simulink model "xieboduoji_13fangzhennow"  (R2023a)
settings: Solver=ode4  StartTime=0.0  StopTime=2.2  FixedStep=5e-7  RelTol=1e-3
undefined symbols (not defined in the file or in its folder): magnitude
libraries: simulink x417, spsRMSLib x70, spsCurrentMeasurementLib x32, spsVoltageMeasurementLib x31, powerlib_meascontrol x24, spsFourierLib x21, spsGroundLib x19, spsThreePhasePISectionLineLib x17, spsThreePhaseSeriesRLCBranchLib x14, spsdq0toAlphaBetaZeroLib x13, spsSeriesRLCBranchLib x11, spsUniversalBridgeLib x11
(part 5 of 12)

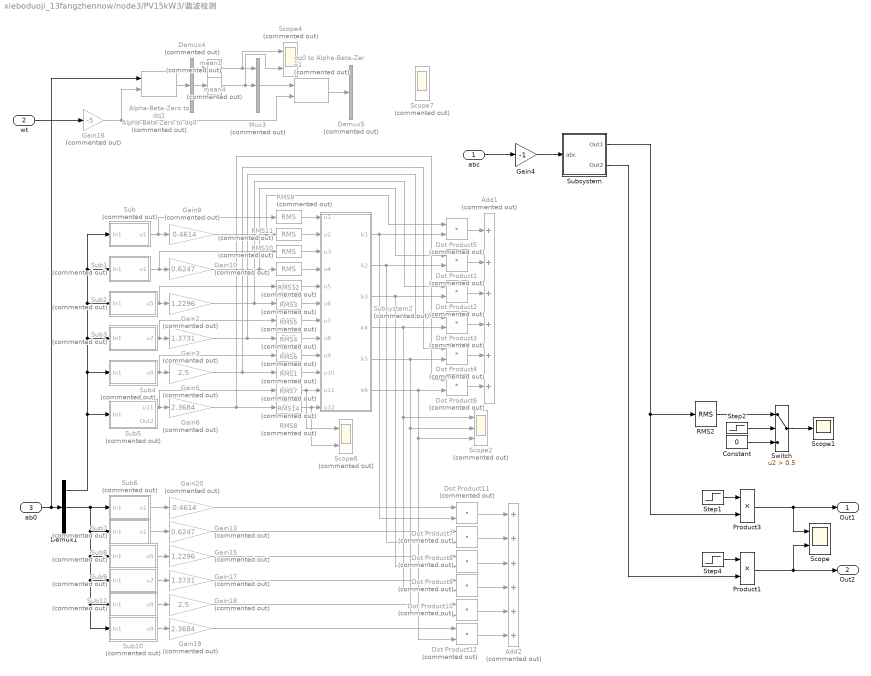
== system xieboduoji_13fangzhennow/node3/PV15kW3/谐波检测 ==
  abc : Inport
  wt : Inport  Port=2
  ab0 : Inport  Port=3
  Add1 : Sum  Commented=on  Inputs=++++++
  Add2 : Sum  Commented=on  Inputs=++++++
  Alpha-Beta-Zero to dq1 : spsAlphaBetaZerotodq0Lib/Alpha-Beta-Zero to dq0  Commented=on  Alignment=Aligned with phase A axis
  Constant : Constant  Value=0
  Demux1 : Demux  Outputs=3
  Demux4 : Demux  Commented=on  Outputs=3
  Demux5 : Demux  Commented=on  Outputs=3
  Dot Product{1..12} (12 alike) : DotProduct  Commented=on  OutDataTypeStr=Inherit: Inherit via internal rule
  Gain10 : Gain  Commented=on  Gain=0.6247
  Gain13 : Gain  Commented=on  Gain=0.6247
  Gain15 : Gain  Commented=on  Gain=1.2296
  Gain16 : Gain  Commented=on  Gain=-5
  Gain17 : Gain  Commented=on  Gain=1.3731
  Gain18 : Gain  Commented=on  Gain=2.5
  Gain19 : Gain  Commented=on  Gain=2.3684
  Gain2 : Gain  Commented=on  Gain=1.2296
  Gain20 : Gain  Commented=on  Gain=0.4614
  Gain3 : Gain  Commented=on  Gain=1.3731
  Gain4 : Gain  Gain=-1
  Gain5 : Gain  Commented=on  Gain=2.5
  Gain6 : Gain  Commented=on  Gain=2.3684
  Gain9 : Gain  Commented=on  Gain=0.4614
  Mux3 : Mux  Commented=on  Inputs=3
  Product1 : Product
  Product3 : Product
  RMS{1,3..12,14} (12 alike) : spsRMSLib/RMS  Commented=on  TrueRMS=on  Freq=100  RMSInit=0  Ts=5e-5
  RMS2 : spsRMSLib/RMS  TrueRMS=on  Freq=50  RMSInit=0  Ts=5e-5
  Scope : Scope  NumInputPorts=2
  Scope1 : Scope
  Scope2 : Scope  Commented=on  NumInputPorts=3
  Scope4 : Scope  Commented=on  NumInputPorts=2
  Scope6 : Scope  Commented=on  NumInputPorts=2
  Scope7 : Scope  Commented=on  NumInputPorts=2
  Step1 : Step  After=-1  SampleTime=0
  Step2 : Step  SampleTime=0
  Step4 : Step  After=-1  SampleTime=0
  Sub : Subsystem  Commented=on
  Sub1 : Subsystem  Commented=on
  Sub10 : Subsystem  Commented=on
  Sub12 : Subsystem  Commented=on
  Sub2 : Subsystem  Commented=on
  Sub3 : Subsystem  Commented=on
  Sub4 : Subsystem  Commented=on
  Sub5 : Subsystem  Commented=on
  Sub6 : Subsystem  Commented=on
  Sub7 : Subsystem  Commented=on
  Sub8 : Subsystem  Commented=on
  Sub9 : Subsystem  Commented=on
  Subsystem : Subsystem
  Subsystem2 : Subsystem  Commented=on
  Switch : Switch  Criteria=u2 > Threshold  Threshold=0.5  SaturateOnIntegerOverflow=off  InputSameDT=off
  dq0 to Alpha-Beta-Zero1 : spsdq0toAlphaBetaZeroLib/dq0 to Alpha-Beta-Zero  Commented=on  Alignment=Aligned with phase A axis
  mean1 : spsMeanLib/Mean  Commented=on  Freq=50  Vinit=0  Ts=5e-5
  mean4 : spsMeanLib/Mean  Commented=on  Freq=50  Vinit=0  Ts=5e-5
  Out1 : Outport
  Out2 : Outport  Port=2
  wires:
  abc/1 -> Gain4/1
  Step1/1 -> Product3/1
  Step2/1 -> Switch/2
  Constant/1 -> Switch/3
  Switch/1 -> Scope1/1
  Sub5/1(u11) -> RMS14/1, Gain6/1
  Sub4/1(u9) -> Gain5/1, RMS1/1
  Sub3/1(u7) -> RMS4/1, Gain3/1
  Sub2/1(u5) -> RMS3/1, Gain2/1
  Demux1/1 -> Sub/1(In1), Sub1/1(In1), Sub2/1(In1), Sub3/1(In1), Sub4/1(In1), Sub5/1(In1)
  Sub1/1(u1) -> RMS10/1, Gain10/1
  Subsystem2/1(k1) -> Dot Product5/2, Dot Product11/2
  Subsystem2/2(k2) -> Dot Product7/2, Dot Product1/2
  Subsystem2/3(k3) -> Dot Product8/2, Dot Product2/2
  Subsystem2/4(k4) -> Scope2/1, Dot Product9/2, Dot Product3/2
  Subsystem2/5(k5) -> Dot Product10/2, Scope2/2, Dot Product4/2
  Sub8/1(u5) -> Gain15/1
  Sub9/1(u7) -> Gain17/1
  Sub12/1(u9) -> Gain18/1
  Demux1/2 -> Sub6/1(In1), Sub7/1(In1), Sub8/1(In1), Sub9/1(In1), Sub10/1(In1), Sub12/1(In1)
  Dot Product12/1 -> Add2/6
  Dot Product10/1 -> Add2/5
  Gain9/1 -> RMS11/1, Dot Product5/1
  Gain2/1 -> RMS5/1, Dot Product2/1
  Gain3/1 -> Dot Product3/1, RMS6/1
  Gain5/1 -> RMS7/1, Dot Product4/1
  Gain6/1 -> Dot Product6/1, RMS8/1
  Gain20/1 -> Dot Product11/1
  Gain13/1 -> Dot Product7/1
  Gain15/1 -> Dot Product8/1
  Gain17/1 -> Dot Product9/1
  Gain18/1 -> Dot Product10/1
  Gain19/1 -> Dot Product12/1
  RMS2/1 -> Switch/1
  RMS7/1 -> Subsystem2/10(u10)
  RMS8/1 -> Scope6/2, Subsystem2/12(u12)
  Gain10/1 -> RMS12/1, Dot Product1/1
  RMS1/1 -> Subsystem2/9(u9)
  RMS14/1 -> Subsystem2/11(u11), Scope6/1
  Dot Product6/1 -> Add1/6
  Dot Product4/1 -> Add1/5
  RMS10/1 -> Subsystem2/3(u3)
  RMS3/1 -> Subsystem2/5(u5)
  RMS5/1 -> Subsystem2/6(u6)
  RMS4/1 -> Subsystem2/7(u7)
  RMS6/1 -> Subsystem2/8(u8)
  Step4/1 -> Product1/1
  Product1/1 -> Scope/2, Out2/1
  Product3/1 -> Scope/1, Out1/1
  Dot Product2/1 -> Add1/3
  Dot Product3/1 -> Add1/4
  Subsystem2/6(k6) -> Scope2/3, Dot Product12/2, Dot Product6/2
  Dot Product8/1 -> Add2/3
  Dot Product9/1 -> Add2/4
  RMS9/1 -> Subsystem2/1(u1)
  Dot Product5/1 -> Add1/1
  Dot Product1/1 -> Add1/2
  Dot Product11/1 -> Add2/1
  Dot Product7/1 -> Add2/2
  RMS11/1 -> Subsystem2/2(u2)
  RMS12/1 -> Subsystem2/4(u4)
  mean1/1 -> Mux3/2, Scope4/2
  mean4/1 -> Mux3/1, Scope4/1
  dq0 to Alpha-Beta-Zero1/1 -> Demux5/1
  Mux3/1 -> dq0 to Alpha-Beta-Zero1/1
  Demux4/2 -> mean1/1
  Demux4/1 -> mean4/1
  Alpha-Beta-Zero to dq1/1 -> Demux4/1
  wt/1 -> Gain16/1
  Gain16/1 -> Alpha-Beta-Zero to dq1/2, dq0 to Alpha-Beta-Zero1/2
  ab0/1 -> Alpha-Beta-Zero to dq1/1, Demux1/1
  Sub/1(u1) -> RMS9/1, Gain9/1
  Sub6/1(u1) -> Gain20/1
  Sub7/1(u1) -> Gain13/1
  Sub10/1(u9) -> Gain19/1
  Gain4/1 -> Subsystem/1(abc)
  Subsystem/1(Out1) -> RMS2/1, Product3/2
  Subsystem/2(Out2) -> Product1/2

== system xieboduoji_13fangzhennow/node3/Subsystem1/RMS1 ==
  u1 : Inport
  u3 : Inport  Port=2
  u4 : Inport  Port=3
  u5 : Inport  Port=4
  u6 : Inport  Port=5
  u2 : Inport  Port=6
  Trigger : TriggerPort  VariantControl=(inherit)
  Scope : Scope  Commented=on
  Scope1 : Scope  Commented=on
  xunidiandao : MATLAB Function  TreatAsAtomicUnit=on
  k1 : Outport  VectorParamsAs1DForOutWhenUnconnected=off
  k2 : Outport  Port=2  VectorParamsAs1DForOutWhenUnconnected=off
  k3 : Outport  Port=3  VectorParamsAs1DForOutWhenUnconnected=off
  k4 : Outport  Port=4  VectorParamsAs1DForOutWhenUnconnected=off
  k5 : Outport  Port=5  VectorParamsAs1DForOutWhenUnconnected=off
  k6 : Outport  Port=6  VectorParamsAs1DForOutWhenUnconnected=off
  k7 : Outport  Port=7  VectorParamsAs1DForOutWhenUnconnected=off
  k8 : Outport  Port=8  VectorParamsAs1DForOutWhenUnconnected=off
  k9 : Outport  Port=9  VectorParamsAs1DForOutWhenUnconnected=off
  k10 : Outport  Port=10  VectorParamsAs1DForOutWhenUnconnected=off
  k11 : Outport  Port=11  VectorParamsAs1DForOutWhenUnconnected=off
  k12 : Outport  Port=12  VectorParamsAs1DForOutWhenUnconnected=off
  wires:
  xunidiandao/13(x) -> Scope/1
  u3/1 -> xunidiandao/2(u2)
  u4/1 -> xunidiandao/3(u3)
  u5/1 -> xunidiandao/4(u4)
  u6/1 -> xunidiandao/5(u5)
  u2/1 -> xunidiandao/6(u6)
  u1/1 -> xunidiandao/1(u1)
  xunidiandao/12(y66) -> k12/1
  xunidiandao/11(y6) -> k11/1
  xunidiandao/10(y55) -> k10/1
  xunidiandao/9(y5) -> k9/1
  xunidiandao/8(y44) -> k8/1
  xunidiandao/7(y4) -> k7/1
  xunidiandao/6(y33) -> k6/1
  xunidiandao/5(y3) -> k5/1
  xunidiandao/4(y22) -> k4/1
  xunidiandao/3(y2) -> k3/1
  xunidiandao/2(y11) -> k2/1
  xunidiandao/1(y1) -> k1/1, Scope1/1

== system xieboduoji_13fangzhennow/node3/Subsystem2/RMS1 ==
  u1 : Inport
  u3 : Inport  Port=2
  u4 : Inport  Port=3
  u5 : Inport  Port=4
  u6 : Inport  Port=5
  u2 : Inport  Port=6
  Trigger : TriggerPort  VariantControl=(inherit)
  Scope : Scope  Commented=on
  Scope1 : Scope  Commented=on
  xunidiandao : MATLAB Function  TreatAsAtomicUnit=on
  k1 : Outport  VectorParamsAs1DForOutWhenUnconnected=off
  k2 : Outport  Port=2  VectorParamsAs1DForOutWhenUnconnected=off
  k3 : Outport  Port=3  VectorParamsAs1DForOutWhenUnconnected=off
  k4 : Outport  Port=4  VectorParamsAs1DForOutWhenUnconnected=off
  k5 : Outport  Port=5  VectorParamsAs1DForOutWhenUnconnected=off
  k6 : Outport  Port=6  VectorParamsAs1DForOutWhenUnconnected=off
  k7 : Outport  Port=7  VectorParamsAs1DForOutWhenUnconnected=off
  k8 : Outport  Port=8  VectorParamsAs1DForOutWhenUnconnected=off
  k9 : Outport  Port=9  VectorParamsAs1DForOutWhenUnconnected=off
  k10 : Outport  Port=10  VectorParamsAs1DForOutWhenUnconnected=off
  k11 : Outport  Port=11  VectorParamsAs1DForOutWhenUnconnected=off
  k12 : Outport  Port=12  VectorParamsAs1DForOutWhenUnconnected=off
  wires:
  xunidiandao/1(y1) -> Scope1/1, k1/1
  xunidiandao/2(y11) -> k2/1
  xunidiandao/3(y2) -> k3/1
  xunidiandao/4(y22) -> k4/1
  xunidiandao/5(y3) -> k5/1
  xunidiandao/6(y33) -> k6/1
  xunidiandao/7(y4) -> k7/1
  xunidiandao/8(y44) -> k8/1
  xunidiandao/9(y5) -> k9/1
  xunidiandao/10(y55) -> k10/1
  xunidiandao/11(y6) -> k11/1
  xunidiandao/12(y66) -> k12/1
  u1/1 -> xunidiandao/1(u1)
  u2/1 -> xunidiandao/6(u6)
  u6/1 -> xunidiandao/5(u5)
  u5/1 -> xunidiandao/4(u4)
  u4/1 -> xunidiandao/3(u3)
  u3/1 -> xunidiandao/2(u2)
  xunidiandao/13(x) -> Scope/1

== system xieboduoji_13fangzhennow/node3/谐波源/Subsystem1 ==
  u1 : Inport
  u3 : Inport  Port=2
  u4 : Inport  Port=3
  u5 : Inport  Port=4
  u6 : Inport  Port=5
  u2 : Inport  Port=6
  Pul : DiscretePulseGenerator  PulseType=Time based  Period=5e-5  PulseWidth=40
  RMS1 : Subsystem  TreatAsAtomicUnit=on
  k1 : Outport  VectorParamsAs1DForOutWhenUnconnected=off
  k2 : Outport  Port=2  VectorParamsAs1DForOutWhenUnconnected=off
  k3 : Outport  Port=3  VectorParamsAs1DForOutWhenUnconnected=off
  k4 : Outport  Port=4  VectorParamsAs1DForOutWhenUnconnected=off
  k5 : Outport  Port=5  VectorParamsAs1DForOutWhenUnconnected=off
  k6 : Outport  Port=6  VectorParamsAs1DForOutWhenUnconnected=off
  k7 : Outport  Port=7  VectorParamsAs1DForOutWhenUnconnected=off
  k8 : Outport  Port=8  VectorParamsAs1DForOutWhenUnconnected=off
  k9 : Outport  Port=9  VectorParamsAs1DForOutWhenUnconnected=off
  k10 : Outport  Port=10  VectorParamsAs1DForOutWhenUnconnected=off
  k11 : Outport  Port=11  VectorParamsAs1DForOutWhenUnconnected=off
  k12 : Outport  Port=12  VectorParamsAs1DForOutWhenUnconnected=off
  wires:
  u2/1 -> RMS1/6(u2)
  u6/1 -> RMS1/5(u6)
  u5/1 -> RMS1/4(u5)
  u4/1 -> RMS1/3(u4)
  u3/1 -> RMS1/2(u3)
  u1/1 -> RMS1/1(u1)
  RMS1/12(k12) -> k12/1
  RMS1/11(k11) -> k11/1
  RMS1/10(k10) -> k10/1
  RMS1/9(k9) -> k9/1
  RMS1/8(k8) -> k8/1
  RMS1/7(k7) -> k7/1
  RMS1/6(k6) -> k6/1
  RMS1/5(k5) -> k5/1
  RMS1/4(k4) -> k4/1
  RMS1/3(k3) -> k3/1
  RMS1/2(k2) -> k2/1
  RMS1/1(k1) -> k1/1
  Pul/1 -> RMS1/Trigger

== system xieboduoji_13fangzhennow/node3/谐波源/Subsystem2 ==
  u1 : Inport
  u3 : Inport  Port=2
  u4 : Inport  Port=3
  u5 : Inport  Port=4
  u6 : Inport  Port=5
  u2 : Inport  Port=6
  Pul : DiscretePulseGenerator  PulseType=Time based  Period=5e-5  PulseWidth=40
  RMS1 : Subsystem  TreatAsAtomicUnit=on
  k1 : Outport  VectorParamsAs1DForOutWhenUnconnected=off
  k2 : Outport  Port=2  VectorParamsAs1DForOutWhenUnconnected=off
  k3 : Outport  Port=3  VectorParamsAs1DForOutWhenUnconnected=off
  k4 : Outport  Port=4  VectorParamsAs1DForOutWhenUnconnected=off
  k5 : Outport  Port=5  VectorParamsAs1DForOutWhenUnconnected=off
  k6 : Outport  Port=6  VectorParamsAs1DForOutWhenUnconnected=off
  k7 : Outport  Port=7  VectorParamsAs1DForOutWhenUnconnected=off
  k8 : Outport  Port=8  VectorParamsAs1DForOutWhenUnconnected=off
  k9 : Outport  Port=9  VectorParamsAs1DForOutWhenUnconnected=off
  k10 : Outport  Port=10  VectorParamsAs1DForOutWhenUnconnected=off
  k11 : Outport  Port=11  VectorParamsAs1DForOutWhenUnconnected=off
  k12 : Outport  Port=12  VectorParamsAs1DForOutWhenUnconnected=off
  wires:
  Pul/1 -> RMS1/Trigger
  RMS1/1(k1) -> k1/1
  RMS1/2(k2) -> k2/1
  RMS1/3(k3) -> k3/1
  RMS1/4(k4) -> k4/1
  RMS1/5(k5) -> k5/1
  RMS1/6(k6) -> k6/1
  RMS1/7(k7) -> k7/1
  RMS1/8(k8) -> k8/1
  RMS1/9(k9) -> k9/1
  RMS1/10(k10) -> k10/1
  RMS1/11(k11) -> k11/1
  RMS1/12(k12) -> k12/1
  u1/1 -> RMS1/1(u1)
  u3/1 -> RMS1/2(u3)
  u4/1 -> RMS1/3(u4)
  u5/1 -> RMS1/4(u5)
  u6/1 -> RMS1/5(u6)
  u2/1 -> RMS1/6(u2)

== system xieboduoji_13fangzhennow/node4/Subsystem1/RMS1 ==
  u1 : Inport
  u3 : Inport  Port=2
  u4 : Inport  Port=3
  u5 : Inport  Port=4
  u6 : Inport  Port=5
  u2 : Inport  Port=6
  Trigger : TriggerPort  VariantControl=(inherit)
  Scope : Scope  Commented=on
  Scope1 : Scope  Commented=on
  xunidiandao : MATLAB Function  TreatAsAtomicUnit=on
  k1 : Outport  VectorParamsAs1DForOutWhenUnconnected=off
  k2 : Outport  Port=2  VectorParamsAs1DForOutWhenUnconnected=off
  k3 : Outport  Port=3  VectorParamsAs1DForOutWhenUnconnected=off
  k4 : Outport  Port=4  VectorParamsAs1DForOutWhenUnconnected=off
  k5 : Outport  Port=5  VectorParamsAs1DForOutWhenUnconnected=off
  k6 : Outport  Port=6  VectorParamsAs1DForOutWhenUnconnected=off
  k7 : Outport  Port=7  VectorParamsAs1DForOutWhenUnconnected=off
  k8 : Outport  Port=8  VectorParamsAs1DForOutWhenUnconnected=off
  k9 : Outport  Port=9  VectorParamsAs1DForOutWhenUnconnected=off
  k10 : Outport  Port=10  VectorParamsAs1DForOutWhenUnconnected=off
  k11 : Outport  Port=11  VectorParamsAs1DForOutWhenUnconnected=off
  k12 : Outport  Port=12  VectorParamsAs1DForOutWhenUnconnected=off
  wires:
  xunidiandao/13(x) -> Scope/1
  u3/1 -> xunidiandao/2(u2)
  u4/1 -> xunidiandao/3(u3)
  u5/1 -> xunidiandao/4(u4)
  u6/1 -> xunidiandao/5(u5)
  u2/1 -> xunidiandao/6(u6)
  u1/1 -> xunidiandao/1(u1)
  xunidiandao/12(y66) -> k12/1
  xunidiandao/11(y6) -> k11/1
  xunidiandao/10(y55) -> k10/1
  xunidiandao/9(y5) -> k9/1
  xunidiandao/8(y44) -> k8/1
  xunidiandao/7(y4) -> k7/1
  xunidiandao/6(y33) -> k6/1
  xunidiandao/5(y3) -> k5/1
  xunidiandao/4(y22) -> k4/1
  xunidiandao/3(y2) -> k3/1
  xunidiandao/2(y11) -> k2/1
  xunidiandao/1(y1) -> k1/1, Scope1/1

== system xieboduoji_13fangzhennow/node4/Subsystem2/RMS1 ==
  u1 : Inport
  u3 : Inport  Port=2
  u4 : Inport  Port=3
  u5 : Inport  Port=4
  u6 : Inport  Port=5
  u2 : Inport  Port=6
  Trigger : TriggerPort  VariantControl=(inherit)
  Scope : Scope  Commented=on
  Scope1 : Scope  Commented=on
  xunidiandao : MATLAB Function  TreatAsAtomicUnit=on
  k1 : Outport  VectorParamsAs1DForOutWhenUnconnected=off
  k2 : Outport  Port=2  VectorParamsAs1DForOutWhenUnconnected=off
  k3 : Outport  Port=3  VectorParamsAs1DForOutWhenUnconnected=off
  k4 : Outport  Port=4  VectorParamsAs1DForOutWhenUnconnected=off
  k5 : Outport  Port=5  VectorParamsAs1DForOutWhenUnconnected=off
  k6 : Outport  Port=6  VectorParamsAs1DForOutWhenUnconnected=off
  k7 : Outport  Port=7  VectorParamsAs1DForOutWhenUnconnected=off
  k8 : Outport  Port=8  VectorParamsAs1DForOutWhenUnconnected=off
  k9 : Outport  Port=9  VectorParamsAs1DForOutWhenUnconnected=off
  k10 : Outport  Port=10  VectorParamsAs1DForOutWhenUnconnected=off
  k11 : Outport  Port=11  VectorParamsAs1DForOutWhenUnconnected=off
  k12 : Outport  Port=12  VectorParamsAs1DForOutWhenUnconnected=off
  wires:
  xunidiandao/1(y1) -> Scope1/1, k1/1
  xunidiandao/2(y11) -> k2/1
  xunidiandao/3(y2) -> k3/1
  xunidiandao/4(y22) -> k4/1
  xunidiandao/5(y3) -> k5/1
  xunidiandao/6(y33) -> k6/1
  xunidiandao/7(y4) -> k7/1
  xunidiandao/8(y44) -> k8/1
  xunidiandao/9(y5) -> k9/1
  xunidiandao/10(y55) -> k10/1
  xunidiandao/11(y6) -> k11/1
  xunidiandao/12(y66) -> k12/1
  u1/1 -> xunidiandao/1(u1)
  u2/1 -> xunidiandao/6(u6)
  u6/1 -> xunidiandao/5(u5)
  u5/1 -> xunidiandao/4(u4)
  u4/1 -> xunidiandao/3(u3)
  u3/1 -> xunidiandao/2(u2)
  xunidiandao/13(x) -> Scope/1

== system xieboduoji_13fangzhennow/node4/谐波源/Subsystem1 ==
  u1 : Inport
  u3 : Inport  Port=2
  u4 : Inport  Port=3
  u5 : Inport  Port=4
  u6 : Inport  Port=5
  u2 : Inport  Port=6
  Pul : DiscretePulseGenerator  PulseType=Time based  Period=5e-5  PulseWidth=40
  RMS1 : Subsystem  TreatAsAtomicUnit=on
  k1 : Outport  VectorParamsAs1DForOutWhenUnconnected=off
  k2 : Outport  Port=2  VectorParamsAs1DForOutWhenUnconnected=off
  k3 : Outport  Port=3  VectorParamsAs1DForOutWhenUnconnected=off
  k4 : Outport  Port=4  VectorParamsAs1DForOutWhenUnconnected=off
  k5 : Outport  Port=5  VectorParamsAs1DForOutWhenUnconnected=off
  k6 : Outport  Port=6  VectorParamsAs1DForOutWhenUnconnected=off
  k7 : Outport  Port=7  VectorParamsAs1DForOutWhenUnconnected=off
  k8 : Outport  Port=8  VectorParamsAs1DForOutWhenUnconnected=off
  k9 : Outport  Port=9  VectorParamsAs1DForOutWhenUnconnected=off
  k10 : Outport  Port=10  VectorParamsAs1DForOutWhenUnconnected=off
  k11 : Outport  Port=11  VectorParamsAs1DForOutWhenUnconnected=off
  k12 : Outport  Port=12  VectorParamsAs1DForOutWhenUnconnected=off
  wires:
  u2/1 -> RMS1/6(u2)
  u6/1 -> RMS1/5(u6)
  u5/1 -> RMS1/4(u5)
  u4/1 -> RMS1/3(u4)
  u3/1 -> RMS1/2(u3)
  u1/1 -> RMS1/1(u1)
  RMS1/12(k12) -> k12/1
  RMS1/11(k11) -> k11/1
  RMS1/10(k10) -> k10/1
  RMS1/9(k9) -> k9/1
  RMS1/8(k8) -> k8/1
  RMS1/7(k7) -> k7/1
  RMS1/6(k6) -> k6/1
  RMS1/5(k5) -> k5/1
  RMS1/4(k4) -> k4/1
  RMS1/3(k3) -> k3/1
  RMS1/2(k2) -> k2/1
  RMS1/1(k1) -> k1/1
  Pul/1 -> RMS1/Trigger

== system xieboduoji_13fangzhennow/node4/谐波源/Subsystem2 ==
  u1 : Inport
  u3 : Inport  Port=2
  u4 : Inport  Port=3
  u5 : Inport  Port=4
  u6 : Inport  Port=5
  u2 : Inport  Port=6
  Pul : DiscretePulseGenerator  PulseType=Time based  Period=5e-5  PulseWidth=40
  RMS1 : Subsystem  TreatAsAtomicUnit=on
  k1 : Outport  VectorParamsAs1DForOutWhenUnconnected=off
  k2 : Outport  Port=2  VectorParamsAs1DForOutWhenUnconnected=off
  k3 : Outport  Port=3  VectorParamsAs1DForOutWhenUnconnected=off
  k4 : Outport  Port=4  VectorParamsAs1DForOutWhenUnconnected=off
  k5 : Outport  Port=5  VectorParamsAs1DForOutWhenUnconnected=off
  k6 : Outport  Port=6  VectorParamsAs1DForOutWhenUnconnected=off
  k7 : Outport  Port=7  VectorParamsAs1DForOutWhenUnconnected=off
  k8 : Outport  Port=8  VectorParamsAs1DForOutWhenUnconnected=off
  k9 : Outport  Port=9  VectorParamsAs1DForOutWhenUnconnected=off
  k10 : Outport  Port=10  VectorParamsAs1DForOutWhenUnconnected=off
  k11 : Outport  Port=11  VectorParamsAs1DForOutWhenUnconnected=off
  k12 : Outport  Port=12  VectorParamsAs1DForOutWhenUnconnected=off
  wires:
  Pul/1 -> RMS1/Trigger
  RMS1/1(k1) -> k1/1
  RMS1/2(k2) -> k2/1
  RMS1/3(k3) -> k3/1
  RMS1/4(k4) -> k4/1
  RMS1/5(k5) -> k5/1
  RMS1/6(k6) -> k6/1
  RMS1/7(k7) -> k7/1
  RMS1/8(k8) -> k8/1
  RMS1/9(k9) -> k9/1
  RMS1/10(k10) -> k10/1
  RMS1/11(k11) -> k11/1
  RMS1/12(k12) -> k12/1
  u1/1 -> RMS1/1(u1)
  u3/1 -> RMS1/2(u3)
  u4/1 -> RMS1/3(u4)
  u5/1 -> RMS1/4(u5)
  u6/1 -> RMS1/5(u6)
  u2/1 -> RMS1/6(u2)

== system xieboduoji_13fangzhennow/node5/Subsystem1/RMS1 ==
  u1 : Inport
  u3 : Inport  Port=2
  u4 : Inport  Port=3
  u5 : Inport  Port=4
  u6 : Inport  Port=5
  u2 : Inport  Port=6
  Trigger : TriggerPort  VariantControl=(inherit)
  Scope : Scope  Commented=on
  Scope1 : Scope  Commented=on
  xunidiandao : MATLAB Function  TreatAsAtomicUnit=on
  k1 : Outport  VectorParamsAs1DForOutWhenUnconnected=off
  k2 : Outport  Port=2  VectorParamsAs1DForOutWhenUnconnected=off
  k3 : Outport  Port=3  VectorParamsAs1DForOutWhenUnconnected=off
  k4 : Outport  Port=4  VectorParamsAs1DForOutWhenUnconnected=off
  k5 : Outport  Port=5  VectorParamsAs1DForOutWhenUnconnected=off
  k6 : Outport  Port=6  VectorParamsAs1DForOutWhenUnconnected=off
  k7 : Outport  Port=7  VectorParamsAs1DForOutWhenUnconnected=off
  k8 : Outport  Port=8  VectorParamsAs1DForOutWhenUnconnected=off
  k9 : Outport  Port=9  VectorParamsAs1DForOutWhenUnconnected=off
  k10 : Outport  Port=10  VectorParamsAs1DForOutWhenUnconnected=off
  k11 : Outport  Port=11  VectorParamsAs1DForOutWhenUnconnected=off
  k12 : Outport  Port=12  VectorParamsAs1DForOutWhenUnconnected=off
  wires:
  xunidiandao/13(x) -> Scope/1
  u3/1 -> xunidiandao/2(u2)
  u4/1 -> xunidiandao/3(u3)
  u5/1 -> xunidiandao/4(u4)
  u6/1 -> xunidiandao/5(u5)
  u2/1 -> xunidiandao/6(u6)
  u1/1 -> xunidiandao/1(u1)
  xunidiandao/12(y66) -> k12/1
  xunidiandao/11(y6) -> k11/1
  xunidiandao/10(y55) -> k10/1
  xunidiandao/9(y5) -> k9/1
  xunidiandao/8(y44) -> k8/1
  xunidiandao/7(y4) -> k7/1
  xunidiandao/6(y33) -> k6/1
  xunidiandao/5(y3) -> k5/1
  xunidiandao/4(y22) -> k4/1
  xunidiandao/3(y2) -> k3/1
  xunidiandao/2(y11) -> k2/1
  xunidiandao/1(y1) -> k1/1, Scope1/1

== system xieboduoji_13fangzhennow/node5/Subsystem2/RMS1 ==
  u1 : Inport
  u3 : Inport  Port=2
  u4 : Inport  Port=3
  u5 : Inport  Port=4
  u6 : Inport  Port=5
  u2 : Inport  Port=6
  Trigger : TriggerPort  VariantControl=(inherit)
  Scope : Scope  Commented=on
  Scope1 : Scope  Commented=on
  xunidiandao : MATLAB Function  TreatAsAtomicUnit=on
  k1 : Outport  VectorParamsAs1DForOutWhenUnconnected=off
  k2 : Outport  Port=2  VectorParamsAs1DForOutWhenUnconnected=off
  k3 : Outport  Port=3  VectorParamsAs1DForOutWhenUnconnected=off
  k4 : Outport  Port=4  VectorParamsAs1DForOutWhenUnconnected=off
  k5 : Outport  Port=5  VectorParamsAs1DForOutWhenUnconnected=off
  k6 : Outport  Port=6  VectorParamsAs1DForOutWhenUnconnected=off
  k7 : Outport  Port=7  VectorParamsAs1DForOutWhenUnconnected=off
  k8 : Outport  Port=8  VectorParamsAs1DForOutWhenUnconnected=off
  k9 : Outport  Port=9  VectorParamsAs1DForOutWhenUnconnected=off
  k10 : Outport  Port=10  VectorParamsAs1DForOutWhenUnconnected=off
  k11 : Outport  Port=11  VectorParamsAs1DForOutWhenUnconnected=off
  k12 : Outport  Port=12  VectorParamsAs1DForOutWhenUnconnected=off
  wires:
  xunidiandao/1(y1) -> Scope1/1, k1/1
  xunidiandao/2(y11) -> k2/1
  xunidiandao/3(y2) -> k3/1
  xunidiandao/4(y22) -> k4/1
  xunidiandao/5(y3) -> k5/1
  xunidiandao/6(y33) -> k6/1
  xunidiandao/7(y4) -> k7/1
  xunidiandao/8(y44) -> k8/1
  xunidiandao/9(y5) -> k9/1
  xunidiandao/10(y55) -> k10/1
  xunidiandao/11(y6) -> k11/1
  xunidiandao/12(y66) -> k12/1
  u1/1 -> xunidiandao/1(u1)
  u2/1 -> xunidiandao/6(u6)
  u6/1 -> xunidiandao/5(u5)
  u5/1 -> xunidiandao/4(u4)
  u4/1 -> xunidiandao/3(u3)
  u3/1 -> xunidiandao/2(u2)
  xunidiandao/13(x) -> Scope/1

== system xieboduoji_13fangzhennow/node5/谐波源/Subsystem1 ==
  u1 : Inport
  u3 : Inport  Port=2
  u4 : Inport  Port=3
  u5 : Inport  Port=4
  u6 : Inport  Port=5
  u2 : Inport  Port=6
  Pul : DiscretePulseGenerator  PulseType=Time based  Period=5e-5  PulseWidth=40
  RMS1 : Subsystem  TreatAsAtomicUnit=on
  k1 : Outport  VectorParamsAs1DForOutWhenUnconnected=off
  k2 : Outport  Port=2  VectorParamsAs1DForOutWhenUnconnected=off
  k3 : Outport  Port=3  VectorParamsAs1DForOutWhenUnconnected=off
  k4 : Outport  Port=4  VectorParamsAs1DForOutWhenUnconnected=off
  k5 : Outport  Port=5  VectorParamsAs1DForOutWhenUnconnected=off
  k6 : Outport  Port=6  VectorParamsAs1DForOutWhenUnconnected=off
  k7 : Outport  Port=7  VectorParamsAs1DForOutWhenUnconnected=off
  k8 : Outport  Port=8  VectorParamsAs1DForOutWhenUnconnected=off
  k9 : Outport  Port=9  VectorParamsAs1DForOutWhenUnconnected=off
  k10 : Outport  Port=10  VectorParamsAs1DForOutWhenUnconnected=off
  k11 : Outport  Port=11  VectorParamsAs1DForOutWhenUnconnected=off
  k12 : Outport  Port=12  VectorParamsAs1DForOutWhenUnconnected=off
  wires:
  u2/1 -> RMS1/6(u2)
  u6/1 -> RMS1/5(u6)
  u5/1 -> RMS1/4(u5)
  u4/1 -> RMS1/3(u4)
  u3/1 -> RMS1/2(u3)
  u1/1 -> RMS1/1(u1)
  RMS1/12(k12) -> k12/1
  RMS1/11(k11) -> k11/1
  RMS1/10(k10) -> k10/1
  RMS1/9(k9) -> k9/1
  RMS1/8(k8) -> k8/1
  RMS1/7(k7) -> k7/1
  RMS1/6(k6) -> k6/1
  RMS1/5(k5) -> k5/1
  RMS1/4(k4) -> k4/1
  RMS1/3(k3) -> k3/1
  RMS1/2(k2) -> k2/1
  RMS1/1(k1) -> k1/1
  Pul/1 -> RMS1/Trigger

== system xieboduoji_13fangzhennow/node5/谐波源/Subsystem2 ==
  u1 : Inport
  u3 : Inport  Port=2
  u4 : Inport  Port=3
  u5 : Inport  Port=4
  u6 : Inport  Port=5
  u2 : Inport  Port=6
  Pul : DiscretePulseGenerator  PulseType=Time based  Period=5e-5  PulseWidth=40
  RMS1 : Subsystem  TreatAsAtomicUnit=on
  k1 : Outport  VectorParamsAs1DForOutWhenUnconnected=off
  k2 : Outport  Port=2  VectorParamsAs1DForOutWhenUnconnected=off
  k3 : Outport  Port=3  VectorParamsAs1DForOutWhenUnconnected=off
  k4 : Outport  Port=4  VectorParamsAs1DForOutWhenUnconnected=off
  k5 : Outport  Port=5  VectorParamsAs1DForOutWhenUnconnected=off
  k6 : Outport  Port=6  VectorParamsAs1DForOutWhenUnconnected=off
  k7 : Outport  Port=7  VectorParamsAs1DForOutWhenUnconnected=off
  k8 : Outport  Port=8  VectorParamsAs1DForOutWhenUnconnected=off
  k9 : Outport  Port=9  VectorParamsAs1DForOutWhenUnconnected=off
  k10 : Outport  Port=10  VectorParamsAs1DForOutWhenUnconnected=off
  k11 : Outport  Port=11  VectorParamsAs1DForOutWhenUnconnected=off
  k12 : Outport  Port=12  VectorParamsAs1DForOutWhenUnconnected=off
  wires:
  Pul/1 -> RMS1/Trigger
  RMS1/1(k1) -> k1/1
  RMS1/2(k2) -> k2/1
  RMS1/3(k3) -> k3/1
  RMS1/4(k4) -> k4/1
  RMS1/5(k5) -> k5/1
  RMS1/6(k6) -> k6/1
  RMS1/7(k7) -> k7/1
  RMS1/8(k8) -> k8/1
  RMS1/9(k9) -> k9/1
  RMS1/10(k10) -> k10/1
  RMS1/11(k11) -> k11/1
  RMS1/12(k12) -> k12/1
  u1/1 -> RMS1/1(u1)
  u3/1 -> RMS1/2(u3)
  u4/1 -> RMS1/3(u4)
  u5/1 -> RMS1/4(u5)
  u6/1 -> RMS1/5(u6)
  u2/1 -> RMS1/6(u2)

== system xieboduoji_13fangzhennow/node8/Subsystem1/RMS1 ==
  u1 : Inport
  u3 : Inport  Port=2
  u4 : Inport  Port=3
  u5 : Inport  Port=4
  u6 : Inport  Port=5
  u2 : Inport  Port=6
  Trigger : TriggerPort  VariantControl=(inherit)
  Scope : Scope  Commented=on
  Scope1 : Scope  Commented=on
  xunidiandao : MATLAB Function  TreatAsAtomicUnit=on
  k1 : Outport  VectorParamsAs1DForOutWhenUnconnected=off
  k2 : Outport  Port=2  VectorParamsAs1DForOutWhenUnconnected=off
  k3 : Outport  Port=3  VectorParamsAs1DForOutWhenUnconnected=off
  k4 : Outport  Port=4  VectorParamsAs1DForOutWhenUnconnected=off
  k5 : Outport  Port=5  VectorParamsAs1DForOutWhenUnconnected=off
  k6 : Outport  Port=6  VectorParamsAs1DForOutWhenUnconnected=off
  k7 : Outport  Port=7  VectorParamsAs1DForOutWhenUnconnected=off
  k8 : Outport  Port=8  VectorParamsAs1DForOutWhenUnconnected=off
  k9 : Outport  Port=9  VectorParamsAs1DForOutWhenUnconnected=off
  k10 : Outport  Port=10  VectorParamsAs1DForOutWhenUnconnected=off
  k11 : Outport  Port=11  VectorParamsAs1DForOutWhenUnconnected=off
  k12 : Outport  Port=12  VectorParamsAs1DForOutWhenUnconnected=off
  wires:
  xunidiandao/13(x) -> Scope/1
  u3/1 -> xunidiandao/2(u2)
  u4/1 -> xunidiandao/3(u3)
  u5/1 -> xunidiandao/4(u4)
  u6/1 -> xunidiandao/5(u5)
  u2/1 -> xunidiandao/6(u6)
  u1/1 -> xunidiandao/1(u1)
  xunidiandao/12(y66) -> k12/1
  xunidiandao/11(y6) -> k11/1
  xunidiandao/10(y55) -> k10/1
  xunidiandao/9(y5) -> k9/1
  xunidiandao/8(y44) -> k8/1
  xunidiandao/7(y4) -> k7/1
  xunidiandao/6(y33) -> k6/1
  xunidiandao/5(y3) -> k5/1
  xunidiandao/4(y22) -> k4/1
  xunidiandao/3(y2) -> k3/1
  xunidiandao/2(y11) -> k2/1
  xunidiandao/1(y1) -> k1/1, Scope1/1

== system xieboduoji_13fangzhennow/node8/Subsystem2/RMS1 ==
  u1 : Inport
  u3 : Inport  Port=2
  u4 : Inport  Port=3
  u5 : Inport  Port=4
  u6 : Inport  Port=5
  u2 : Inport  Port=6
  Trigger : TriggerPort  VariantControl=(inherit)
  Scope : Scope  Commented=on
  Scope1 : Scope  Commented=on
  xunidiandao : MATLAB Function  TreatAsAtomicUnit=on
  k1 : Outport  VectorParamsAs1DForOutWhenUnconnected=off
  k2 : Outport  Port=2  VectorParamsAs1DForOutWhenUnconnected=off
  k3 : Outport  Port=3  VectorParamsAs1DForOutWhenUnconnected=off
  k4 : Outport  Port=4  VectorParamsAs1DForOutWhenUnconnected=off
  k5 : Outport  Port=5  VectorParamsAs1DForOutWhenUnconnected=off
  k6 : Outport  Port=6  VectorParamsAs1DForOutWhenUnconnected=off
  k7 : Outport  Port=7  VectorParamsAs1DForOutWhenUnconnected=off
  k8 : Outport  Port=8  VectorParamsAs1DForOutWhenUnconnected=off
  k9 : Outport  Port=9  VectorParamsAs1DForOutWhenUnconnected=off
  k10 : Outport  Port=10  VectorParamsAs1DForOutWhenUnconnected=off
  k11 : Outport  Port=11  VectorParamsAs1DForOutWhenUnconnected=off
  k12 : Outport  Port=12  VectorParamsAs1DForOutWhenUnconnected=off
  wires:
  xunidiandao/1(y1) -> Scope1/1, k1/1
  xunidiandao/2(y11) -> k2/1
  xunidiandao/3(y2) -> k3/1
  xunidiandao/4(y22) -> k4/1
  xunidiandao/5(y3) -> k5/1
  xunidiandao/6(y33) -> k6/1
  xunidiandao/7(y4) -> k7/1
  xunidiandao/8(y44) -> k8/1
  xunidiandao/9(y5) -> k9/1
  xunidiandao/10(y55) -> k10/1
  xunidiandao/11(y6) -> k11/1
  xunidiandao/12(y66) -> k12/1
  u1/1 -> xunidiandao/1(u1)
  u2/1 -> xunidiandao/6(u6)
  u6/1 -> xunidiandao/5(u5)
  u5/1 -> xunidiandao/4(u4)
  u4/1 -> xunidiandao/3(u3)
  u3/1 -> xunidiandao/2(u2)
  xunidiandao/13(x) -> Scope/1

== system xieboduoji_13fangzhennow/node8/谐波源/Subsystem1 ==
  u1 : Inport
  u3 : Inport  Port=2
  u4 : Inport  Port=3
  u5 : Inport  Port=4
  u6 : Inport  Port=5
  u2 : Inport  Port=6
  Pul : DiscretePulseGenerator  PulseType=Time based  Period=5e-5  PulseWidth=40
  RMS1 : Subsystem  TreatAsAtomicUnit=on
  k1 : Outport  VectorParamsAs1DForOutWhenUnconnected=off
  k2 : Outport  Port=2  VectorParamsAs1DForOutWhenUnconnected=off
  k3 : Outport  Port=3  VectorParamsAs1DForOutWhenUnconnected=off
  k4 : Outport  Port=4  VectorParamsAs1DForOutWhenUnconnected=off
  k5 : Outport  Port=5  VectorParamsAs1DForOutWhenUnconnected=off
  k6 : Outport  Port=6  VectorParamsAs1DForOutWhenUnconnected=off
  k7 : Outport  Port=7  VectorParamsAs1DForOutWhenUnconnected=off
  k8 : Outport  Port=8  VectorParamsAs1DForOutWhenUnconnected=off
  k9 : Outport  Port=9  VectorParamsAs1DForOutWhenUnconnected=off
  k10 : Outport  Port=10  VectorParamsAs1DForOutWhenUnconnected=off
  k11 : Outport  Port=11  VectorParamsAs1DForOutWhenUnconnected=off
  k12 : Outport  Port=12  VectorParamsAs1DForOutWhenUnconnected=off
  wires:
  u2/1 -> RMS1/6(u2)
  u6/1 -> RMS1/5(u6)
  u5/1 -> RMS1/4(u5)
  u4/1 -> RMS1/3(u4)
  u3/1 -> RMS1/2(u3)
  u1/1 -> RMS1/1(u1)
  RMS1/12(k12) -> k12/1
  RMS1/11(k11) -> k11/1
  RMS1/10(k10) -> k10/1
  RMS1/9(k9) -> k9/1
  RMS1/8(k8) -> k8/1
  RMS1/7(k7) -> k7/1
  RMS1/6(k6) -> k6/1
  RMS1/5(k5) -> k5/1
  RMS1/4(k4) -> k4/1
  RMS1/3(k3) -> k3/1
  RMS1/2(k2) -> k2/1
  RMS1/1(k1) -> k1/1
  Pul/1 -> RMS1/Trigger

== system xieboduoji_13fangzhennow/node8/谐波源/Subsystem2 ==
  u1 : Inport
  u3 : Inport  Port=2
  u4 : Inport  Port=3
  u5 : Inport  Port=4
  u6 : Inport  Port=5
  u2 : Inport  Port=6
  Pul : DiscretePulseGenerator  PulseType=Time based  Period=5e-5  PulseWidth=40
  RMS1 : Subsystem  TreatAsAtomicUnit=on
  k1 : Outport  VectorParamsAs1DForOutWhenUnconnected=off
  k2 : Outport  Port=2  VectorParamsAs1DForOutWhenUnconnected=off
  k3 : Outport  Port=3  VectorParamsAs1DForOutWhenUnconnected=off
  k4 : Outport  Port=4  VectorParamsAs1DForOutWhenUnconnected=off
  k5 : Outport  Port=5  VectorParamsAs1DForOutWhenUnconnected=off
  k6 : Outport  Port=6  VectorParamsAs1DForOutWhenUnconnected=off
  k7 : Outport  Port=7  VectorParamsAs1DForOutWhenUnconnected=off
  k8 : Outport  Port=8  VectorParamsAs1DForOutWhenUnconnected=off
  k9 : Outport  Port=9  VectorParamsAs1DForOutWhenUnconnected=off
  k10 : Outport  Port=10  VectorParamsAs1DForOutWhenUnconnected=off
  k11 : Outport  Port=11  VectorParamsAs1DForOutWhenUnconnected=off
  k12 : Outport  Port=12  VectorParamsAs1DForOutWhenUnconnected=off
  wires:
  Pul/1 -> RMS1/Trigger
  RMS1/1(k1) -> k1/1
  RMS1/2(k2) -> k2/1
  RMS1/3(k3) -> k3/1
  RMS1/4(k4) -> k4/1
  RMS1/5(k5) -> k5/1
  RMS1/6(k6) -> k6/1
  RMS1/7(k7) -> k7/1
  RMS1/8(k8) -> k8/1
  RMS1/9(k9) -> k9/1
  RMS1/10(k10) -> k10/1
  RMS1/11(k11) -> k11/1
  RMS1/12(k12) -> k12/1
  u1/1 -> RMS1/1(u1)
  u3/1 -> RMS1/2(u3)
  u4/1 -> RMS1/3(u4)
  u5/1 -> RMS1/4(u5)
  u6/1 -> RMS1/5(u6)
  u2/1 -> RMS1/6(u2)

== system xieboduoji_13fangzhennow/node10/谐波源/Subsystem1/RMS1 ==
  u1 : Inport
  u3 : Inport  Port=2
  u4 : Inport  Port=3
  u5 : Inport  Port=4
  u6 : Inport  Port=5
  u2 : Inport  Port=6
  Trigger : TriggerPort  VariantControl=(inherit)
  Scope : Scope  Commented=on
  Scope1 : Scope  Commented=on
  xunidiandao : MATLAB Function  TreatAsAtomicUnit=on
  k1 : Outport  VectorParamsAs1DForOutWhenUnconnected=off
  k2 : Outport  Port=2  VectorParamsAs1DForOutWhenUnconnected=off
  k3 : Outport  Port=3  VectorParamsAs1DForOutWhenUnconnected=off
  k4 : Outport  Port=4  VectorParamsAs1DForOutWhenUnconnected=off
  k5 : Outport  Port=5  VectorParamsAs1DForOutWhenUnconnected=off
  k6 : Outport  Port=6  VectorParamsAs1DForOutWhenUnconnected=off
  k7 : Outport  Port=7  VectorParamsAs1DForOutWhenUnconnected=off
  k8 : Outport  Port=8  VectorParamsAs1DForOutWhenUnconnected=off
  k9 : Outport  Port=9  VectorParamsAs1DForOutWhenUnconnected=off
  k10 : Outport  Port=10  VectorParamsAs1DForOutWhenUnconnected=off
  k11 : Outport  Port=11  VectorParamsAs1DForOutWhenUnconnected=off
  k12 : Outport  Port=12  VectorParamsAs1DForOutWhenUnconnected=off
  wires:
  xunidiandao/13(x) -> Scope/1
  u3/1 -> xunidiandao/2(u2)
  u4/1 -> xunidiandao/3(u3)
  u5/1 -> xunidiandao/4(u4)
  u6/1 -> xunidiandao/5(u5)
  u2/1 -> xunidiandao/6(u6)
  u1/1 -> xunidiandao/1(u1)
  xunidiandao/12(y66) -> k12/1
  xunidiandao/11(y6) -> k11/1
  xunidiandao/10(y55) -> k10/1
  xunidiandao/9(y5) -> k9/1
  xunidiandao/8(y44) -> k8/1
  xunidiandao/7(y4) -> k7/1
  xunidiandao/6(y33) -> k6/1
  xunidiandao/5(y3) -> k5/1
  xunidiandao/4(y22) -> k4/1
  xunidiandao/3(y2) -> k3/1
  xunidiandao/2(y11) -> k2/1
  xunidiandao/1(y1) -> k1/1, Scope1/1

== system xieboduoji_13fangzhennow/node10/谐波源/Subsystem2/RMS1 ==
  u1 : Inport
  u3 : Inport  Port=2
  u4 : Inport  Port=3
  u5 : Inport  Port=4
  u6 : Inport  Port=5
  u2 : Inport  Port=6
  Trigger : TriggerPort  VariantControl=(inherit)
  Scope : Scope  Commented=on
  Scope1 : Scope  Commented=on
  xunidiandao : MATLAB Function  TreatAsAtomicUnit=on
  k1 : Outport  VectorParamsAs1DForOutWhenUnconnected=off
  k2 : Outport  Port=2  VectorParamsAs1DForOutWhenUnconnected=off
  k3 : Outport  Port=3  VectorParamsAs1DForOutWhenUnconnected=off
  k4 : Outport  Port=4  VectorParamsAs1DForOutWhenUnconnected=off
  k5 : Outport  Port=5  VectorParamsAs1DForOutWhenUnconnected=off
  k6 : Outport  Port=6  VectorParamsAs1DForOutWhenUnconnected=off
  k7 : Outport  Port=7  VectorParamsAs1DForOutWhenUnconnected=off
  k8 : Outport  Port=8  VectorParamsAs1DForOutWhenUnconnected=off
  k9 : Outport  Port=9  VectorParamsAs1DForOutWhenUnconnected=off
  k10 : Outport  Port=10  VectorParamsAs1DForOutWhenUnconnected=off
  k11 : Outport  Port=11  VectorParamsAs1DForOutWhenUnconnected=off
  k12 : Outport  Port=12  VectorParamsAs1DForOutWhenUnconnected=off
  wires:
  xunidiandao/1(y1) -> Scope1/1, k1/1
  xunidiandao/2(y11) -> k2/1
  xunidiandao/3(y2) -> k3/1
  xunidiandao/4(y22) -> k4/1
  xunidiandao/5(y3) -> k5/1
  xunidiandao/6(y33) -> k6/1
  xunidiandao/7(y4) -> k7/1
  xunidiandao/8(y44) -> k8/1
  xunidiandao/9(y5) -> k9/1
  xunidiandao/10(y55) -> k10/1
  xunidiandao/11(y6) -> k11/1
  xunidiandao/12(y66) -> k12/1
  u1/1 -> xunidiandao/1(u1)
  u2/1 -> xunidiandao/6(u6)
  u6/1 -> xunidiandao/5(u5)
  u5/1 -> xunidiandao/4(u4)
  u4/1 -> xunidiandao/3(u3)
  u3/1 -> xunidiandao/2(u2)
  xunidiandao/13(x) -> Scope/1

== system xieboduoji_13fangzhennow/node12/PV15kW3/PWM2/PWM3 ==
  In1 : Inport
  Abs : Abs  SaturateOnIntegerOverflow=off
  Abs1 : Abs  SaturateOnIntegerOverflow=off
  Abs2 : Abs  SaturateOnIntegerOverflow=off
  Bus Creator1 : BusCreator  Inputs=6
  Constant : Constant
  Data Type Conversion{,1..5} (6 alike) : DataTypeConversion  OutDataTypeStr=double  SaturateOnIntegerOverflow=off  RndMeth=Floor
  Delay : Delay  DelayLength=4  InitialCondition=0
  Delay1 : Delay  DelayLength=4  InitialCondition=0
  Delay2 : Delay  DelayLength=4  InitialCondition=0
  Demux1 : Demux  Outputs=3
  Logical Operator : Logic  Operator=NOT  AllPortsSameDT=off  OutDataTypeStr=boolean
  Logical Operator1 : Logic  Operator=NOT  AllPortsSameDT=off  OutDataTypeStr=boolean
  Logical Operator2 : Logic  Operator=NOT  AllPortsSameDT=off  OutDataTypeStr=boolean
  Product{,1..5} (6 alike) : Product
  Relational Operator : RelationalOperator  OutDataTypeStr=boolean  InputSameDT=off
  Relational Operator1 : RelationalOperator  OutDataTypeStr=boolean  InputSameDT=off
  Relational Operator2 : RelationalOperator  OutDataTypeStr=boolean  InputSameDT=off
  Repeating Sequence : simulink/Sources/Repeating Sequence  rep_seq_t=[0 0.5*0.5e-4 0.5*1e-4]  rep_seq_y=[0 2 0]
  Sum : Sum  Inputs=|++
  Sum1 : Sum  Inputs=+-
  Sum2 : Sum  Inputs=+-
  Sum3 : Sum  Inputs=+-
  switch : Outport  PortDimensions=6  VectorParamsAs1DForOutWhenUnconnected=off
  Out1 : Outport  Port=2  VectorParamsAs1DForOutWhenUnconnected=off
  wires:
  Relational Operator2/1 -> Data Type Conversion4/1, Logical Operator2/1
  Demux1/3 -> Relational Operator2/1
  Relational Operator1/1 -> Data Type Conversion2/1, Logical Operator1/1
  Demux1/2 -> Relational Operator1/1
  Logical Operator/1 -> Data Type Conversion1/1
  Relational Operator/1 -> Logical Operator/1, Data Type Conversion/1
  Demux1/1 -> Relational Operator/1
  Sum/1 -> Out1/1, Demux1/1
  In1/1 -> Sum/2
  Constant/1 -> Sum/1
  Repeating Sequence/1 -> Relational Operator2/2, Relational Operator1/2, Relational Operator/2
  Bus Creator1/1 -> switch/1
  Data Type Conversion/1 -> Product/1, Sum1/1
  Data Type Conversion1/1 -> Delay/1
  Delay/1 -> Sum1/2, Product1/2
  Sum1/1 -> Abs/1
  Product/1 -> Bus Creator1/1
  Abs/1 -> Product/2, Product1/1
  Product1/1 -> Bus Creator1/2
  Abs1/1 -> Product3/1, Product2/2
  Sum2/1 -> Abs1/1
  Delay1/1 -> Product3/2, Sum2/2
  Data Type Conversion3/1 -> Delay1/1
  Data Type Conversion2/1 -> Product2/1, Sum2/1
  Data Type Conversion4/1 -> Sum3/1, Product4/1
  Data Type Conversion5/1 -> Delay2/1
  Delay2/1 -> Sum3/2, Product5/2
  Sum3/1 -> Abs2/1
  Abs2/1 -> Product4/2, Product5/1
  Logical Operator1/1 -> Data Type Conversion3/1
  Logical Operator2/1 -> Data Type Conversion5/1
  Product4/1 -> Bus Creator1/5
  Product5/1 -> Bus Creator1/6
  Product3/1 -> Bus Creator1/4
  Product2/1 -> Bus Creator1/3

== system xieboduoji_13fangzhennow/node12/PV15kW3/Subsystem9/integral  ==
  di : Inport
  Trigger : TriggerPort  VariantControl=(inherit)
  Embedded MATLAB Function : MATLAB Function  TreatAsAtomicUnit=on
  w : Outport
  wires:
  Embedded MATLAB Function/1(w) -> w/1
  di/1 -> Embedded MATLAB Function/1(er)

== system xieboduoji_13fangzhennow/node12/PV15kW3/改进PLL1/PI ==
  Vgq : Inport
  Trigger : TriggerPort  VariantControl=(inherit)
  Embedded MATLAB Function : MATLAB Function  TreatAsAtomicUnit=on
  w : Outport  VectorParamsAs1DForOutWhenUnconnected=off
  wires:
  Embedded MATLAB Function/1(w) -> w/1
  Vgq/1 -> Embedded MATLAB Function/1(Vgq)

== system xieboduoji_13fangzhennow/node12/PV15kW3/改进PLL1/Subsystem2 ==
  In1 : Inport
  Demux6 : Demux  Outputs=3
  Discrete Transfer Fcn1 : DiscreteTransferFcn  Commented=on  Numerator=[-0.984414127416096 1]  Denominator=[1 -0.984414127416096]  SampleTime=5e-5
  Discrete Transfer Fcn4 : DiscreteTransferFcn  Commented=on  Numerator=[0.004690094552539 0 -0.004690094552539]  Denominator=[1 -1.990374233068895 0.990619810894922]  SampleTime=5e-5
  Mux5 : Mux  Inputs=3
  SOGI滤波50Hz2 : TransferFcn  Numerator=[0.6*100*pi 0]  Denominator=[1 0.6*100*pi 10000*pi*pi]
  SOGI滤波50Hz3 : TransferFcn  Numerator=[0.6*100*pi 0]  Denominator=[1 0.6*100*pi 10000*pi*pi]
  Terminator : Terminator
  Out1 : Outport
  wires:
  SOGI滤波50Hz3/1 -> Mux5/1  "alpha"
  Demux6/3 -> Terminator/1
  In1/1 -> Demux6/1
  Demux6/2 -> SOGI滤波50Hz2/1
  Mux5/1 -> Out1/1
  Demux6/1 -> SOGI滤波50Hz3/1
  SOGI滤波50Hz2/1 -> Mux5/2  "belta"

== system xieboduoji_13fangzhennow/node12/PV15kW3/谐波检测/Sub1 ==
  In1 : Inport
  Constant1 : Constant  Value=-60*pi/180
  Constant{10,12,15,17} (4 alike) : Constant  Value=100*pi
  Constant11 : Constant  Value=5
  Constant2 : Constant  Value=-60*pi/180
  Cos : Trigonometry  Operator=cos
  Cos1 : Trigonometry  Operator=cos
  Cos2 : Trigonometry
  Cos3 : Trigonometry
  Delay : Delay  DelayLength=400  SampleTime=5e-5
  Delay1 : Delay  DelayLength=1  SampleTime=5e-5
  Delay2 : Delay  DelayLength=1  SampleTime=5e-5
  Divide{,1..3} (4 alike) : Product  Inputs=***
  Dot Product{,1..2,4} (4 alike) : DotProduct  OutDataTypeStr=Inherit: Inherit via internal rule
  Gain : Gain  Gain=2/400
  Gain10 : Gain  Gain=2/400
  Ramp{,1..3} (4 alike) : simulink/Sources/Ramp  slope=1  start=0  InitialOutput=0
  Sum{,1,3,9,18} (5 alike) : Sum  Inputs=|++
  Sum2 : Sum  Inputs=-+|
  u1 : Outport
  wires:
  [thk] -> Divide/1
  Constant11/1 -> [thk]
  Sum9/1 -> u1/1
  Dot Product1/1 -> Sum9/1
  Gain/1 -> Sum3/1
  Ramp2/1 -> Divide2/3
  Constant10/1 -> Divide/2
  Delay2/1 -> Sum18/2
  Gain10/1 -> Sum18/1
  Sum3/1 -> Delay1/1, Dot Product1/2
  Delay/1 -> Sum2/1
  Ramp1/1 -> Divide1/3
  Constant12/1 -> Divide1/2
  Divide2/1 -> Cos2/1
  Cos3/1 -> Dot Product4/2
  Dot Product2/1 -> Gain10/1
  Cos2/1 -> Dot Product2/2
  Delay1/1 -> Sum3/2
  Ramp3/1 -> Divide3/3
  [thk] -> Divide1/1
  Dot Product4/1 -> Sum9/2
  [thk] -> Divide2/1
  [thk] -> Divide3/1
  Sum18/1 -> Delay2/1, Dot Product4/1
  Constant15/1 -> Divide2/2
  In1/1 -> Sum2/2, Delay/1
  Dot Product/1 -> Gain/1
  Cos/1 -> Dot Product/1
  Divide/1 -> Cos/1
  Sum2/1 -> Dot Product/2, Dot Product2/1
  Ramp/1 -> Divide/3
  Constant17/1 -> Divide3/2
  Cos1/1 -> Dot Product1/1
  Divide1/1 -> Sum/1
  Sum/1 -> Cos1/1
  Sum1/1 -> Cos3/1
  Divide3/1 -> Sum1/1

== system xieboduoji_13fangzhennow/node12/PV15kW3/谐波检测/Sub10 ==
  In1 : Inport
  Constant{10,12,15,17} (4 alike) : Constant  Value=100*pi
  Constant11 : Constant  Value=17
  Cos : Trigonometry  Operator=cos
  Cos1 : Trigonometry  Operator=cos
  Cos2 : Trigonometry
  Cos3 : Trigonometry
  Delay : Delay  DelayLength=400  SampleTime=5e-5
  Delay1 : Delay  DelayLength=1  SampleTime=5e-5
  Delay2 : Delay  DelayLength=1  SampleTime=5e-5
  Divide{,1..3} (4 alike) : Product  Inputs=***
  Dot Product{,1..2,4} (4 alike) : DotProduct  OutDataTypeStr=Inherit: Inherit via internal rule
  Gain : Gain  Gain=2/400
  Gain10 : Gain  Gain=2/400
  Ramp{,1..3} (4 alike) : simulink/Sources/Ramp  slope=1  start=0  InitialOutput=0
  Sum18 : Sum  Inputs=|++
  Sum2 : Sum  Inputs=-+|
  Sum3 : Sum  Inputs=|++
  Sum9 : Sum  Inputs=|++
  Out1 : Outport
  wires:
  Constant17/1 -> Divide3/2
  Ramp/1 -> Divide/3
  Sum2/1 -> Dot Product2/1, Dot Product/2
  Divide/1 -> Cos/1
  Cos/1 -> Dot Product/1
  Dot Product/1 -> Gain/1
  Cos1/1 -> Dot Product1/1
  In1/1 -> Delay/1, Sum2/2
  Constant15/1 -> Divide2/2
  Sum18/1 -> Dot Product4/1, Delay2/1
  [thk] -> Divide3/1
  [thk] -> Divide2/1
  Dot Product4/1 -> Sum9/2
  [thk] -> Divide1/1
  Ramp3/1 -> Divide3/3
  Divide3/1 -> Cos3/1
  Delay1/1 -> Sum3/2
  Cos2/1 -> Dot Product2/2
  Dot Product2/1 -> Gain10/1
  Cos3/1 -> Dot Product4/2
  Divide2/1 -> Cos2/1
  Constant12/1 -> Divide1/2
  Ramp1/1 -> Divide1/3
  Divide1/1 -> Cos1/1
  Delay/1 -> Sum2/1
  Sum3/1 -> Dot Product1/2, Delay1/1
  Gain10/1 -> Sum18/1
  Delay2/1 -> Sum18/2
  Constant10/1 -> Divide/2
  Ramp2/1 -> Divide2/3
  Gain/1 -> Sum3/1
  Dot Product1/1 -> Sum9/1
  Sum9/1 -> Out1/1
  Constant11/1 -> [thk]
  [thk] -> Divide/1

== system xieboduoji_13fangzhennow/node12/PV15kW3/谐波检测/Sub11 ==
  In1 : Inport
  Constant{10,12,15,17} (4 alike) : Constant  Value=100*pi
  Constant11 : Constant  Value=19
  Cos : Trigonometry  Operator=cos
  Cos1 : Trigonometry  Operator=cos
  Cos2 : Trigonometry
  Cos3 : Trigonometry
  Delay : Delay  DelayLength=400  SampleTime=5e-5
  Delay1 : Delay  DelayLength=1  SampleTime=5e-5
  Delay2 : Delay  DelayLength=1  SampleTime=5e-5
  Divide{,1..3} (4 alike) : Product  Inputs=***
  Dot Product{,1..2,4} (4 alike) : DotProduct  OutDataTypeStr=Inherit: Inherit via internal rule
  Gain : Gain  Gain=2/400
  Gain10 : Gain  Gain=2/400
  Ramp{,1..3} (4 alike) : simulink/Sources/Ramp  slope=1  start=0  InitialOutput=0
  Sum18 : Sum  Inputs=|++
  Sum2 : Sum  Inputs=-+|
  Sum3 : Sum  Inputs=|++
  Sum9 : Sum  Inputs=|++
  Out1 : Outport
  wires:
  [thk] -> Divide/1
  Constant11/1 -> [thk]
  Sum9/1 -> Out1/1
  Dot Product1/1 -> Sum9/1
  Gain/1 -> Sum3/1
  Ramp2/1 -> Divide2/3
  Constant10/1 -> Divide/2
  Delay2/1 -> Sum18/2
  Gain10/1 -> Sum18/1
  Sum3/1 -> Delay1/1, Dot Product1/2
  Delay/1 -> Sum2/1
  Divide1/1 -> Cos1/1
  Ramp1/1 -> Divide1/3
  Constant12/1 -> Divide1/2
  Divide2/1 -> Cos2/1
  Cos3/1 -> Dot Product4/2
  Dot Product2/1 -> Gain10/1
  Cos2/1 -> Dot Product2/2
  Delay1/1 -> Sum3/2
  Divide3/1 -> Cos3/1
  Ramp3/1 -> Divide3/3
  [thk] -> Divide1/1
  Dot Product4/1 -> Sum9/2
  [thk] -> Divide2/1
  [thk] -> Divide3/1
  Sum18/1 -> Delay2/1, Dot Product4/1
  Constant15/1 -> Divide2/2
  In1/1 -> Sum2/2, Delay/1
  Cos1/1 -> Dot Product1/1
  Dot Product/1 -> Gain/1
  Cos/1 -> Dot Product/1
  Divide/1 -> Cos/1
  Sum2/1 -> Dot Product/2, Dot Product2/1
  Ramp/1 -> Divide/3
  Constant17/1 -> Divide3/2

== system xieboduoji_13fangzhennow/node12/PV15kW3/谐波检测/Sub12 ==
  In1 : Inport
  Constant1 : Constant  Value=-60*pi/180
  Constant{10,12,15,17} (4 alike) : Constant  Value=100*pi
  Constant11 : Constant  Value=7
  Constant2 : Constant  Value=-60*pi/180
  Cos : Trigonometry  Operator=cos
  Cos1 : Trigonometry  Operator=cos
  Cos2 : Trigonometry
  Cos3 : Trigonometry
  Delay : Delay  DelayLength=400  SampleTime=5e-5
  Delay1 : Delay  DelayLength=1  SampleTime=5e-5
  Delay2 : Delay  DelayLength=1  SampleTime=5e-5
  Divide{,1..3} (4 alike) : Product  Inputs=***
  Dot Product{,1..2,4} (4 alike) : DotProduct  OutDataTypeStr=Inherit: Inherit via internal rule
  Gain : Gain  Gain=2/400
  Gain10 : Gain  Gain=2/400
  Ramp{,1..3} (4 alike) : simulink/Sources/Ramp  slope=1  start=0  InitialOutput=0
  Sum{,1,3,9,18} (5 alike) : Sum  Inputs=|++
  Sum2 : Sum  Inputs=-+|
  u1 : Outport
  wires:
  Divide3/1 -> Sum1/1
  Sum1/1 -> Cos3/1
  Sum/1 -> Cos1/1
  Divide1/1 -> Sum/1
  Cos1/1 -> Dot Product1/1
  Constant17/1 -> Divide3/2
  Ramp/1 -> Divide/3
  Sum2/1 -> Dot Product2/1, Dot Product/2
  Divide/1 -> Cos/1
  Cos/1 -> Dot Product/1
  Dot Product/1 -> Gain/1
  In1/1 -> Delay/1, Sum2/2
  Constant15/1 -> Divide2/2
  Sum18/1 -> Dot Product4/1, Delay2/1
  [thk] -> Divide3/1
  [thk] -> Divide2/1
  Dot Product4/1 -> Sum9/2
  [thk] -> Divide1/1
  Ramp3/1 -> Divide3/3
  Delay1/1 -> Sum3/2
  Cos2/1 -> Dot Product2/2
  Dot Product2/1 -> Gain10/1
  Cos3/1 -> Dot Product4/2
  Divide2/1 -> Cos2/1
  Constant12/1 -> Divide1/2
  Ramp1/1 -> Divide1/3
  Delay/1 -> Sum2/1
  Sum3/1 -> Dot Product1/2, Delay1/1
  Gain10/1 -> Sum18/1
  Delay2/1 -> Sum18/2
  Constant10/1 -> Divide/2
  Ramp2/1 -> Divide2/3
  Gain/1 -> Sum3/1
  Dot Product1/1 -> Sum9/1
  Sum9/1 -> u1/1
  Constant11/1 -> [thk]
  [thk] -> Divide/1

== system xieboduoji_13fangzhennow/node12/PV15kW3/谐波检测/Sub2 ==
  In1 : Inport
  Constant{10,12,15,17} (4 alike) : Constant  Value=100*pi
  Constant11 : Constant  Value=11
  Cos : Trigonometry  Operator=cos
  Cos1 : Trigonometry  Operator=cos
  Cos2 : Trigonometry
  Cos3 : Trigonometry
  Delay : Delay  DelayLength=400  SampleTime=5e-5
  Delay1 : Delay  DelayLength=1  SampleTime=5e-5
  Delay2 : Delay  DelayLength=1  SampleTime=5e-5
  Divide{,1..3} (4 alike) : Product  Inputs=***
  Dot Product{,1..2,4} (4 alike) : DotProduct  OutDataTypeStr=Inherit: Inherit via internal rule
  Gain : Gain  Gain=2/400
  Gain10 : Gain  Gain=2/400
  Ramp{,1..3} (4 alike) : simulink/Sources/Ramp  slope=1  start=0  InitialOutput=0
  Sum18 : Sum  Inputs=|++
  Sum2 : Sum  Inputs=-+|
  Sum3 : Sum  Inputs=|++
  Sum9 : Sum  Inputs=|++
  u5 : Outport
  wires:
  [thk] -> Divide/1
  Constant11/1 -> [thk]
  Sum9/1 -> u5/1
  Dot Product1/1 -> Sum9/1
  Gain/1 -> Sum3/1
  Ramp2/1 -> Divide2/3
  Constant10/1 -> Divide/2
  Delay2/1 -> Sum18/2
  Gain10/1 -> Sum18/1
  Sum3/1 -> Delay1/1, Dot Product1/2
  Delay/1 -> Sum2/1
  Divide1/1 -> Cos1/1
  Ramp1/1 -> Divide1/3
  Constant12/1 -> Divide1/2
  Divide2/1 -> Cos2/1
  Cos3/1 -> Dot Product4/2
  Dot Product2/1 -> Gain10/1
  Cos2/1 -> Dot Product2/2
  Delay1/1 -> Sum3/2
  Divide3/1 -> Cos3/1
  Ramp3/1 -> Divide3/3
  [thk] -> Divide1/1
  Dot Product4/1 -> Sum9/2
  [thk] -> Divide2/1
  [thk] -> Divide3/1
  Sum18/1 -> Delay2/1, Dot Product4/1
  Constant15/1 -> Divide2/2
  In1/1 -> Sum2/2, Delay/1
  Cos1/1 -> Dot Product1/1
  Dot Product/1 -> Gain/1
  Cos/1 -> Dot Product/1
  Divide/1 -> Cos/1
  Sum2/1 -> Dot Product/2, Dot Product2/1
  Ramp/1 -> Divide/3
  Constant17/1 -> Divide3/2

== system xieboduoji_13fangzhennow/node12/PV15kW3/谐波检测/Sub3 ==
  In1 : Inport
  Constant{10,12,15,17} (4 alike) : Constant  Value=100*pi
  Constant11 : Constant  Value=13
  Cos : Trigonometry  Operator=cos
  Cos1 : Trigonometry  Operator=cos
  Cos2 : Trigonometry
  Cos3 : Trigonometry
  Delay : Delay  DelayLength=400  SampleTime=5e-5
  Delay1 : Delay  DelayLength=1  SampleTime=5e-5
  Delay2 : Delay  DelayLength=1  SampleTime=5e-5
  Divide{,1..3} (4 alike) : Product  Inputs=***
  Dot Product{,1..2,4} (4 alike) : DotProduct  OutDataTypeStr=Inherit: Inherit via internal rule
  Gain : Gain  Gain=2/400
  Gain10 : Gain  Gain=2/400
  Ramp{,1..3} (4 alike) : simulink/Sources/Ramp  slope=1  start=0  InitialOutput=0
  Sum18 : Sum  Inputs=|++
  Sum2 : Sum  Inputs=-+|
  Sum3 : Sum  Inputs=|++
  Sum9 : Sum  Inputs=|++
  u7 : Outport
  wires:
  Constant17/1 -> Divide3/2
  Ramp/1 -> Divide/3
  Sum2/1 -> Dot Product2/1, Dot Product/2
  Divide/1 -> Cos/1
  Cos/1 -> Dot Product/1
  Dot Product/1 -> Gain/1
  Cos1/1 -> Dot Product1/1
  In1/1 -> Delay/1, Sum2/2
  Constant15/1 -> Divide2/2
  Sum18/1 -> Dot Product4/1, Delay2/1
  [thk] -> Divide3/1
  [thk] -> Divide2/1
  Dot Product4/1 -> Sum9/2
  [thk] -> Divide1/1
  Ramp3/1 -> Divide3/3
  Divide3/1 -> Cos3/1
  Delay1/1 -> Sum3/2
  Cos2/1 -> Dot Product2/2
  Dot Product2/1 -> Gain10/1
  Cos3/1 -> Dot Product4/2
  Divide2/1 -> Cos2/1
  Constant12/1 -> Divide1/2
  Ramp1/1 -> Divide1/3
  Divide1/1 -> Cos1/1
  Delay/1 -> Sum2/1
  Sum3/1 -> Dot Product1/2, Delay1/1
  Gain10/1 -> Sum18/1
  Delay2/1 -> Sum18/2
  Constant10/1 -> Divide/2
  Ramp2/1 -> Divide2/3
  Gain/1 -> Sum3/1
  Dot Product1/1 -> Sum9/1
  Sum9/1 -> u7/1
  Constant11/1 -> [thk]
  [thk] -> Divide/1
